simulink model "S200_Simulation"  (R2018b)
settings: Solver=VariableStepAuto  StartTime=0.0  StopTime=100  RelTol=1e-3
values from neighbouring files (symbols this model uses):
  alpha_linear = 0.95    [Parameter_S200_Simulation.m]
  delta_ksi = (5-(-5))/(9-1)    (= 1.25)    [Gaussverteilung.m]    (also in Parameter_S200_Simulation.m = 1.14285714286)
  eta_linear = 10^(-3)    (= 0.001)    [Parameter_S200_Simulation.m]
  h = 10^(-3)    (= 0.001)    [Parameter_S200_Simulation.m]
  J = 0.166    [Parameter_S200_Simulation.m]
  ksi = linspace(-20,20,36)    [Parameter_S200_Simulation.m]
  l = 30    [Parameter_S200_Simulation.m]
  sigma_norm = 1.3    [Parameter_S200_Simulation.m]
undefined symbols (not defined in the file or in its folder): alpha_NL, DiscIntNeverNeededParam, eta_NL
settings Model: Creator=LENOVO  LastModifiedBy=LENOVO

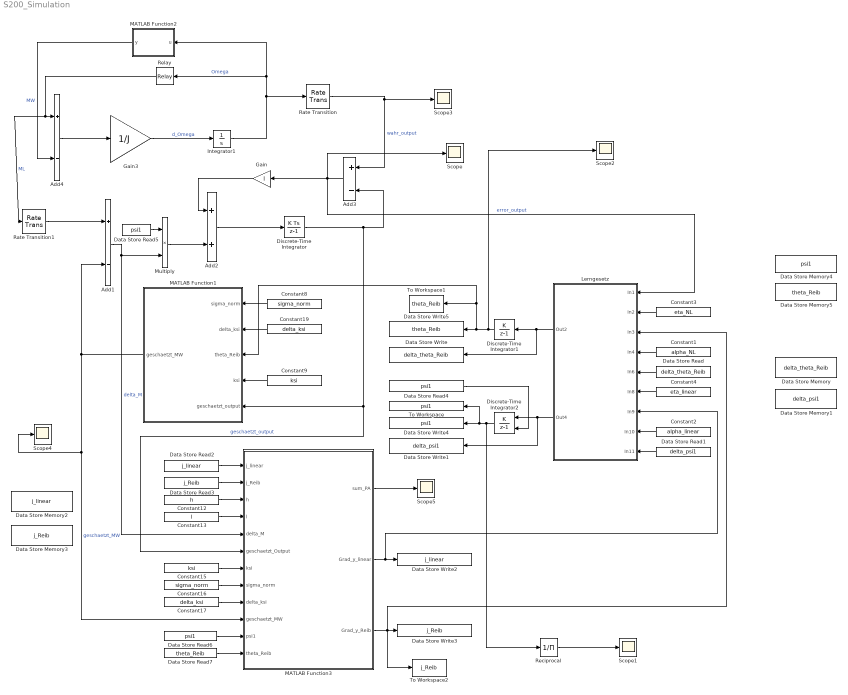
== system S200_Simulation ==
  Add1 : Sum  Inputs=+-
  Add2 : Sum
  Add3 : Sum  Inputs=+-
  Add4 : Sum  Inputs=+-
  Constant1 : Constant  Value=alpha_NL
  Constant12 : Constant  Value=h
  Constant13 : Constant  Value=l
  Constant15 : Constant  Value=ksi
  Constant16 : Constant  Value=sigma_norm
  Constant17 : Constant  Value=delta_ksi
  Constant19 : Constant  Value=delta_ksi
  Constant2 : Constant  Value=alpha_linear
  Constant3 : Constant  Value=eta_NL
  Constant4 : Constant  Value=eta_linear
  Constant8 : Constant  Value=sigma_norm
  Constant9 : Constant  Value=ksi
  Data Store Memory : DataStoreMemory  DataStoreName=delta_theta_Reib  ReadBeforeWriteMsg=warning  WriteAfterWriteMsg=warning  WriteAfterReadMsg=warning  InitialValue=zeros(1,36)  ShowAdditionalParam=off
  Data Store Memory1 : DataStoreMemory  DataStoreName=delta_psi1  ReadBeforeWriteMsg=warning  WriteAfterWriteMsg=warning  WriteAfterReadMsg=warning  ShowAdditionalParam=off
  Data Store Memory2 : DataStoreMemory  DataStoreName=j_linear  ReadBeforeWriteMsg=warning  WriteAfterWriteMsg=warning  WriteAfterReadMsg=warning  ShowAdditionalParam=off
  Data Store Memory3 : DataStoreMemory  DataStoreName=j_Reib  ReadBeforeWriteMsg=warning  WriteAfterWriteMsg=warning  WriteAfterReadMsg=warning  InitialValue=zeros(1,36)  ShowAdditionalParam=off
  Data Store Memory4 : DataStoreMemory  DataStoreName=psi1  ReadBeforeWriteMsg=warning  WriteAfterWriteMsg=warning  WriteAfterReadMsg=warning  InitialValue=5  ShowAdditionalParam=off
  Data Store Memory5 : DataStoreMemory  DataStoreName=theta_Reib  ReadBeforeWriteMsg=warning  WriteAfterWriteMsg=warning  WriteAfterReadMsg=warning  InitialValue=zeros(1,36)  ShowAdditionalParam=off
  Data Store Read : DataStoreRead  DataStoreName=delta_theta_Reib
  Data Store Read1 : DataStoreRead  DataStoreName=delta_psi1
  Data Store Read2 : DataStoreRead  DataStoreName=j_linear
  Data Store Read3 : DataStoreRead  DataStoreName=j_Reib
  Data Store Read4 : DataStoreRead  DataStoreName=psi1
  Data Store Read5 : DataStoreRead  DataStoreName=psi1
  Data Store Read6 : DataStoreRead  DataStoreName=psi1
  Data Store Read7 : DataStoreRead  DataStoreName=theta_Reib
  Data Store Write : DataStoreWrite  DataStoreName=delta_theta_Reib
  Data Store Write1 : DataStoreWrite  DataStoreName=delta_psi1
  Data Store Write2 : DataStoreWrite  DataStoreName=j_linear
  Data Store Write3 : DataStoreWrite  DataStoreName=j_Reib
  Data Store Write4 : DataStoreWrite  DataStoreName=psi1
  Data Store Write5 : DataStoreWrite  DataStoreName=theta_Reib
  Discrete-Time Integrator : DiscreteIntegrator  InitialCondition=-20  SampleTime=-1  UpperSaturationLimit=20  LowerSaturationLimit=-20  ICPrevOutput=DiscIntNeverNeededParam  ICPrevScaledInput=DiscIntNeverNeededParam
  Discrete-Time Integrator1 : DiscreteIntegrator  IntegratorMethod=Accumulation: Forward Euler  gainval=1  SampleTime=-1  ICPrevOutput=DiscIntNeverNeededParam  ICPrevScaledInput=DiscIntNeverNeededParam
  Discrete-Time Integrator2 : DiscreteIntegrator  IntegratorMethod=Accumulation: Forward Euler  gainval=1  InitialConditionSource=external  SampleTime=-1  ICPrevOutput=DiscIntNeverNeededParam  ICPrevScaledInput=DiscIntNeverNeededParam
  Gain : Gain  Gain=l
  Gain3 : Gain  Gain=1/J
  Integrator1 : Integrator  InitialCondition=-20
  Lerngesetz : Subsystem
  MATLAB Function1 : MATLAB Function  TreatAsAtomicUnit=on
  MATLAB Function2 : MATLAB Function  TreatAsAtomicUnit=on
  MATLAB Function3 : MATLAB Function  TreatAsAtomicUnit=on
  Multiply : Product
  Rate Transition : RateTransition  Deterministic=off  OutPortSampleTime=0.001
  Rate Transition1 : RateTransition  OutPortSampleTime=0.001
  Reciprocal : Product  Inputs=/
  Relay : Relay  OnSwitchValue=20  OffSwitchValue=-20  OnOutputValue=-15  OffOutputValue=15  ZeroCross=off
  Scope{,1..5} (6 alike) : Scope
  To Workspace : ToWorkspace  VariableName=psi1  SaveFormat=Timeseries  SampleTime=-1
      settings: Save2DSignal=2-D array (concatenate along first dimension)
  To Workspace1 : ToWorkspace  VariableName=theta_Reib  SampleTime=-1
      settings: Save2DSignal=2-D array (concatenate along first dimension)
  To Workspace2 : ToWorkspace  VariableName=j_Reib  SaveFormat=Timeseries  SampleTime=-1
  wires:
  Rate Transition1/1 -> Add1/1
  Add1/1 -> Multiply/2, MATLAB Function3/5(delta_M)  "delta_M"
  Add2/1 -> Discrete-Time Integrator/1
  Discrete-Time Integrator/1 -> Add3/2, MATLAB Function3/6(geschaetzt_Output), MATLAB Function1/5(geschaetzt_output)  "geschaetzt_output"
  Rate Transition/1 -> Add3/1, Scope3/1  "wahr_output"
  Add3/1 -> Scope/1, Lerngesetz/1(In1), Gain/1  "error_output"
  Gain3/1 -> Integrator1/1  "d_Omega"
  Add4/1 -> Gain3/1
  Integrator1/1 -> Relay/1, MATLAB Function2/1(u), Rate Transition/1  "Omega"
  Relay/1 -> Rate Transition1/1, Add4/1  "ML"
  MATLAB Function2/1(y) -> Add4/2  "MW"
  Constant1/1 -> Lerngesetz/4(In4)
  Constant2/1 -> Lerngesetz/8(In10)
  Constant3/1 -> Lerngesetz/2(In2)
  Data Store Read/1 -> Lerngesetz/5(In6)
  Data Store Read1/1 -> Lerngesetz/9(In11)
  Lerngesetz/2(Out4) -> Discrete-Time Integrator2/1, Data Store Write1/1
  Lerngesetz/1(Out2) -> Discrete-Time Integrator1/1, Data Store Write/1
  MATLAB Function1/1(geschaetzt_MW) -> Scope4/1, MATLAB Function3/10(geschaetzt_MW), Add1/2  "geschaetzt_MW"
  Constant8/1 -> MATLAB Function1/1(sigma_norm)
  Constant9/1 -> MATLAB Function1/4(ksi)
  Data Store Read2/1 -> MATLAB Function3/1(j_linear)
  Data Store Read3/1 -> MATLAB Function3/2(j_Reib)
  Constant12/1 -> MATLAB Function3/3(h)
  Constant13/1 -> MATLAB Function3/4(l)
  Constant15/1 -> MATLAB Function3/7(ksi)
  Constant16/1 -> MATLAB Function3/8(sigma_norm)
  Constant17/1 -> MATLAB Function3/9(delta_ksi)
  MATLAB Function3/2(Grad_y_linear) -> Lerngesetz/7(In9), Data Store Write2/1
  MATLAB Function3/3(Grad_y_Reib) -> Lerngesetz/3(In3), Data Store Write3/1, To Workspace2/1
  Constant19/1 -> MATLAB Function1/2(delta_ksi)
  Constant4/1 -> Lerngesetz/6(In8)
  Discrete-Time Integrator1/1 -> Scope2/1, Data Store Write5/1, To Workspace1/1, MATLAB Function1/3(theta_Reib)
  Discrete-Time Integrator2/1 -> To Workspace/1, Data Store Write4/1, Reciprocal/1
  Data Store Read4/1 -> Discrete-Time Integrator2/2
  Multiply/1 -> Add2/2
  Data Store Read5/1 -> Multiply/1
  Data Store Read6/1 -> MATLAB Function3/11(psi1)
  Data Store Read7/1 -> MATLAB Function3/12(theta_Reib)
  Gain/1 -> Add2/1
  Reciprocal/1 -> Scope1/1
  MATLAB Function3/1(sum_PA) -> Scope5/1

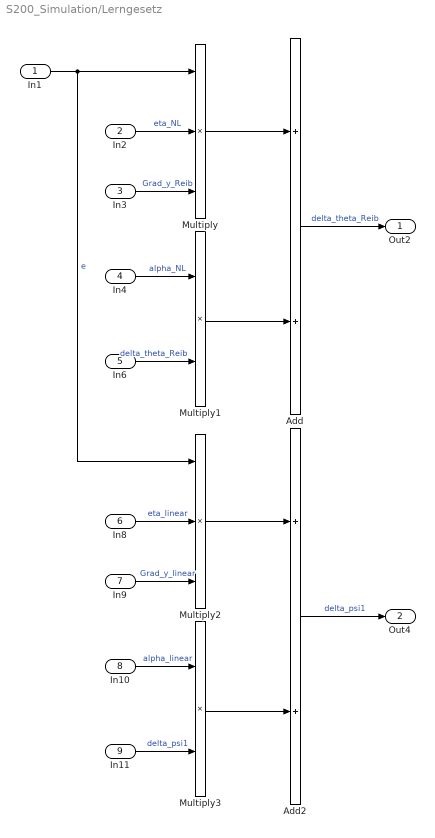
== system S200_Simulation/Lerngesetz ==
  In1 : Inport
  In2 : Inport  Port=2
  In3 : Inport  Port=3
  In4 : Inport  Port=4
  In6 : Inport  Port=5
  In8 : Inport  Port=6
  In9 : Inport  Port=7
  In10 : Inport  Port=8
  In11 : Inport  Port=9
  Add : Sum  Inputs=2
  Add2 : Sum  Inputs=2
  Multiply : Product  Inputs=3
  Multiply1 : Product
  Multiply2 : Product  Inputs=3
  Multiply3 : Product
  Out2 : Outport
  Out4 : Outport  Port=2
  wires:
  In3/1 -> Multiply/3  "Grad_y_Reib"
  In2/1 -> Multiply/2  "eta_NL"
  In1/1 -> Multiply/1, Multiply2/1  "e"
  In4/1 -> Multiply1/1  "alpha_NL"
  In6/1 -> Multiply1/2  "delta_theta_Reib"
  Multiply1/1 -> Add/2
  Multiply/1 -> Add/1
  Add/1 -> Out2/1  "delta_theta_Reib"
  Add2/1 -> Out4/1  "delta_psi1"
  Multiply2/1 -> Add2/1
  Multiply3/1 -> Add2/2
  In11/1 -> Multiply3/2  "delta_psi1"
  In10/1 -> Multiply3/1  "alpha_linear"
  In8/1 -> Multiply2/2  "eta_linear"
  In9/1 -> Multiply2/3  "Grad_y_linear"

== matlab function S200_Simulation/MATLAB Function2 ==
  data: u input; y output
function y = MW(u)

if u>=0
    MW=0.29*atan(0.3*u)+0.4;
else
    MW=0.35*atan(0.3*u)-0.15;
end

y = MW;

end

== matlab function S200_Simulation/MATLAB Function1 ==
  data: sigma_norm input; delta_ksi input; geschaetzt_MW output; theta_Reib input; ksi input; geschaetzt_output input
function geschaetzt_MW=Sum(sigma_norm,delta_ksi,theta_Reib,ksi,geschaetzt_output)

Zaehler_AF_GRNN=@(u,ksi) exp(-(u-ksi).^2/(2*sigma_norm^2*delta_ksi^2));
Nenner_AF_GRNN=@(u,ksi) sum(Zaehler_AF_GRNN(u,ksi));
AF_GRNN=@(u,ksi) Zaehler_AF_GRNN(u,ksi)/Nenner_AF_GRNN(u,ksi); %Aktivierungsfunktionen

geschaetzt_MW=sum(theta_Reib.*AF_GRNN(geschaetzt_output,ksi));

end

== matlab function S200_Simulation/MATLAB Function3 ==
  data: sum_PA output; j_linear input; Grad_y_linear output; j_Reib input; Grad_y_Reib output; h input; l input; delta_M input; geschaetzt_Output input; ksi input; sigma_norm input; delta_ksi input; geschaetzt_MW input; psi1 input; theta_Reib input
function [sum_PA,Grad_y_linear,Grad_y_Reib]=Partielle_Ableitung(j_linear,j_Reib,h,l,delta_M,geschaetzt_Output,ksi,sigma_norm,delta_ksi,geschaetzt_MW,psi1,theta_Reib)

Zaehler_AF_GRNN=@(u,ksi) exp(-(u-ksi).^2/(2*sigma_norm^2*delta_ksi^2));
Nenner_AF_GRNN=@(u,ksi) sum(Zaehler_AF_GRNN(u,ksi));
AF_GRNN=@(u,ksi) Zaehler_AF_GRNN(u,ksi)/Nenner_AF_GRNN(u,ksi); %Aktivierungsfunktionen

sum_PA=0;

for j=1:30
    sum_PA=sum_PA+Zaehler_AF_GRNN(geschaetzt_Output,ksi(j))/Nenner_AF_GRNN(geschaetzt_Output,ksi)*(geschaetzt_Output-ksi(j))/(sigma_norm^2*delta_ksi^2)*(geschaetzt_MW-theta_Reib(j));
end

delta_y_GRNN_linear=j_linear.*sum_PA;
delta_y_GRNN_NL=Zaehler_AF_GRNN(geschaetzt_Output,ksi)/Nenner_AF_GRNN(geschaetzt_Output,ksi)+j_Reib.*sum_PA;

j_linear=(1-h*l)*j_linear+h*delta_M-h*psi1*delta_y_GRNN_linear;
j_Reib=(1-h*l).*j_Reib-h*psi1.*delta_y_GRNN_NL;

Grad_y_linear=j_linear;
Grad_y_Reib=j_Reib;
end
